simulink library "INT_CrCtl_ShOff"  (R2016b)
settings: Solver=VariableStepAuto  StartTime=0.0  StopTime=10.0  RelTol=1e-3
settings Model: Creator=guanxiaoxing  LastModifiedBy=guanxiaoxing

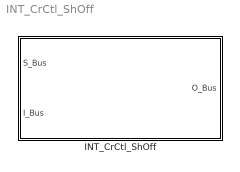
== system INT_CrCtl_ShOff ==
  INT_CrCtl_ShOff : Subsystem

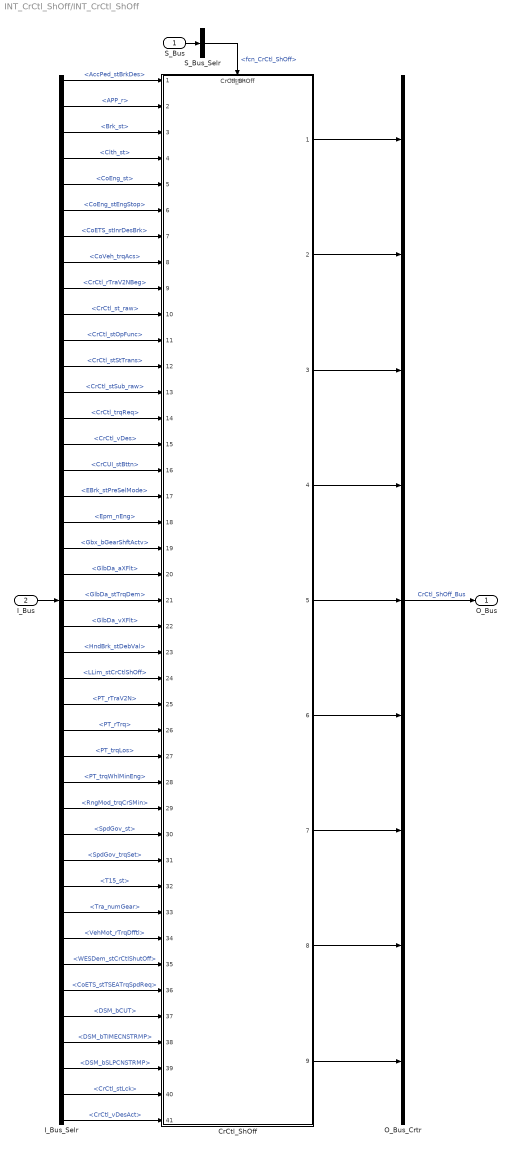
== system INT_CrCtl_ShOff/INT_CrCtl_ShOff ==
  S_Bus : Inport
  I_Bus : Inport  Port=2
  CrCtl_ShOff : ModelReference  ModelNameDialog=CrCtl_ShOff  SimulationMode=Normal  ModelReferenceVersion=1.140  TriggerPortName=function  TriggerPortTriggerType=function-call  TriggerPortStatesWhenEnabling=held
  I_Bus_Selr : BusSelector  OutputSignals=AccPed_stBrkDes,APP_r,Brk_st,Clth_st,CoEng_st,CoEng_stEngStop,CoETS_stInrDesBrk,CoVeh_trqAcs,CrCtl_rTraV2NBeg,CrCtl_st_raw,CrCtl_stOpFunc,CrCtl_stStTrans,CrCtl_stSub_raw,CrCtl_trqReq,CrCtl_vDes,CrCUI_stBttn,EBrk_stPreSelMode,Epm_nEng,Gbx_bGearShftActv,GlbDa_aXFlt,GlbDa_stTrqDem,GlbDa_vXFlt,HndBrk_stDebVal,LLim_stCrCtlShOff,PT_rTraV2N,PT_rTrq,PT_trqLos,PT_trqWhlMinEng,RngMod_trqCrSMin,SpdGov_st,SpdGov_trqSet,T15_st,Tra_numGear,VehMot_rTrqDfftl,WESDem_stCrCtlShutOff,CoETS_stTSEATrqSpdReq,DSM_bCUT,DSM_bTIMECNSTRMP,DSM_bSLPCNSTRMP,CrCtl_stLck,CrCtl_vDesAct
  O_Bus_Crtr : BusCreator  Inputs=9
  S_Bus_Selr : BusSelector  OutputSignals=fcn_CrCtl_ShOff
  O_Bus : Outport
  wires:
  S_Bus_Selr/1 -> CrCtl_ShOff/Trigger  "<fcn_CrCtl_ShOff>"
  S_Bus/1 -> S_Bus_Selr/1
  I_Bus/1 -> I_Bus_Selr/1
  I_Bus_Selr/1 -> CrCtl_ShOff/1  "<AccPed_stBrkDes>"
  I_Bus_Selr/2 -> CrCtl_ShOff/2  "<APP_r>"
  I_Bus_Selr/3 -> CrCtl_ShOff/3  "<Brk_st>"
  I_Bus_Selr/4 -> CrCtl_ShOff/4  "<Clth_st>"
  I_Bus_Selr/5 -> CrCtl_ShOff/5  "<CoEng_st>"
  I_Bus_Selr/6 -> CrCtl_ShOff/6  "<CoEng_stEngStop>"
  I_Bus_Selr/7 -> CrCtl_ShOff/7  "<CoETS_stInrDesBrk>"
  I_Bus_Selr/8 -> CrCtl_ShOff/8  "<CoVeh_trqAcs>"
  I_Bus_Selr/9 -> CrCtl_ShOff/9  "<CrCtl_rTraV2NBeg>"
  I_Bus_Selr/10 -> CrCtl_ShOff/10  "<CrCtl_st_raw>"
  I_Bus_Selr/11 -> CrCtl_ShOff/11  "<CrCtl_stOpFunc>"
  I_Bus_Selr/12 -> CrCtl_ShOff/12  "<CrCtl_stStTrans>"
  I_Bus_Selr/13 -> CrCtl_ShOff/13  "<CrCtl_stSub_raw>"
  I_Bus_Selr/14 -> CrCtl_ShOff/14  "<CrCtl_trqReq>"
  I_Bus_Selr/15 -> CrCtl_ShOff/15  "<CrCtl_vDes>"
  I_Bus_Selr/16 -> CrCtl_ShOff/16  "<CrCUI_stBttn>"
  I_Bus_Selr/17 -> CrCtl_ShOff/17  "<EBrk_stPreSelMode>"
  I_Bus_Selr/18 -> CrCtl_ShOff/18  "<Epm_nEng>"
  I_Bus_Selr/19 -> CrCtl_ShOff/19  "<Gbx_bGearShftActv>"
  I_Bus_Selr/20 -> CrCtl_ShOff/20  "<GlbDa_aXFlt>"
  I_Bus_Selr/21 -> CrCtl_ShOff/21  "<GlbDa_stTrqDem>"
  I_Bus_Selr/22 -> CrCtl_ShOff/22  "<GlbDa_vXFlt>"
  I_Bus_Selr/23 -> CrCtl_ShOff/23  "<HndBrk_stDebVal>"
  I_Bus_Selr/24 -> CrCtl_ShOff/24  "<LLim_stCrCtlShOff>"
  I_Bus_Selr/25 -> CrCtl_ShOff/25  "<PT_rTraV2N>"
  I_Bus_Selr/26 -> CrCtl_ShOff/26  "<PT_rTrq>"
  I_Bus_Selr/27 -> CrCtl_ShOff/27  "<PT_trqLos>"
  I_Bus_Selr/28 -> CrCtl_ShOff/28  "<PT_trqWhlMinEng>"
  I_Bus_Selr/29 -> CrCtl_ShOff/29  "<RngMod_trqCrSMin>"
  I_Bus_Selr/30 -> CrCtl_ShOff/30  "<SpdGov_st>"
  I_Bus_Selr/31 -> CrCtl_ShOff/31  "<SpdGov_trqSet>"
  I_Bus_Selr/32 -> CrCtl_ShOff/32  "<T15_st>"
  I_Bus_Selr/33 -> CrCtl_ShOff/33  "<Tra_numGear>"
  I_Bus_Selr/34 -> CrCtl_ShOff/34  "<VehMot_rTrqDfftl>"
  I_Bus_Selr/35 -> CrCtl_ShOff/35  "<WESDem_stCrCtlShutOff>"
  I_Bus_Selr/36 -> CrCtl_ShOff/36  "<CoETS_stTSEATrqSpdReq>"
  I_Bus_Selr/37 -> CrCtl_ShOff/37  "<DSM_bCUT>"
  I_Bus_Selr/38 -> CrCtl_ShOff/38  "<DSM_bTIMECNSTRMP>"
  I_Bus_Selr/39 -> CrCtl_ShOff/39  "<DSM_bSLPCNSTRMP>"
  I_Bus_Selr/40 -> CrCtl_ShOff/40  "<CrCtl_stLck>"
  I_Bus_Selr/41 -> CrCtl_ShOff/41  "<CrCtl_vDesAct>"
  O_Bus_Crtr/1 -> O_Bus/1  "CrCtl_ShOff_Bus"
  CrCtl_ShOff/1 -> O_Bus_Crtr/1
  CrCtl_ShOff/2 -> O_Bus_Crtr/2
  CrCtl_ShOff/3 -> O_Bus_Crtr/3
  CrCtl_ShOff/4 -> O_Bus_Crtr/4
  CrCtl_ShOff/5 -> O_Bus_Crtr/5
  CrCtl_ShOff/6 -> O_Bus_Crtr/6
  CrCtl_ShOff/7 -> O_Bus_Crtr/7
  CrCtl_ShOff/8 -> O_Bus_Crtr/8
  CrCtl_ShOff/9 -> O_Bus_Crtr/9
